simulink model "CostFunctionTuning"  (R2025b)
settings: Solver=FixedStepAuto  StartTime=0.0  StopTime=10.0  FixedStep=0.5  RelTol=1e-3  EnableMultiTasking=on
undefined symbols (not defined in the file): finalPose, initialPose, samplingBoxCenterPose, samplingBoxDimension, verticesStaticObstacles
libraries: MPSV x3
settings Model: Creator=Scythe  LastModifiedBy=Scythe
settings SolverCC: ConcurrentTasks=on
settings DataIOCC: SaveOutput=off  SignalLogging=off  DSMLogging=off  SaveTime=off  ReturnWorkspaceOutputs=off
settings OptimizationCC: DefaultParameterBehavior=Inlined  ZeroExternalMemoryAtStartup=off  ZeroInternalMemoryAtStartup=off  SimCompilerOptimization=on
settings DebuggingCC: UnconnectedInputMsg=warning  UnconnectedOutputMsg=warning  UnconnectedLineMsg=warning
settings HardwareCC: ProdBitPerLong=64.0  ProdHWDeviceType=Intel->x86-64 (Linux 64)  TargetBitPerLong=64.0  TargetBitPerPointer=64.0  TargetBitPerSizeT=64.0  TargetBitPerPtrDiffT=64.0  TargetLargestAtomicFloat=Float  TargetIntDivRoundTo=Zero  TargetEndianess=LittleEndian  TargetWordSize=64.0  TargetHWDeviceType=Intel->x86-64 (Linux 64)  ProdEqTarget=off
settings ModelReferenceCC: EnableRefExpFcnMdlSchedulingChecks=on
settings SFSimCC: SimParseCustomCode=off  SimGenImportedTypeDefs=on  SimTargetLang=C++  SimDLTargetLibrary=mkl-dnn
settings RTWCC: GenCodeOnly=on  PackageGeneratedCodeAndArtifacts=on  PackageName=PackNGo  BuildConfiguration=Faster Runs  TargetLang=C++
settings CodeAppCC: ForceParamTrailComments=on  MaxIdLength=128.0  StateflowObjectComments=on  MATLABSourceComments=on  UseSimReservedNames=on
settings GRTTargetCC: TargetLangStandard=C++11 (ISO)  MatFileLogging=off  CodeInterfacePackaging=C++ class  SubcomponentCodeInterfacePackaging=C++ class

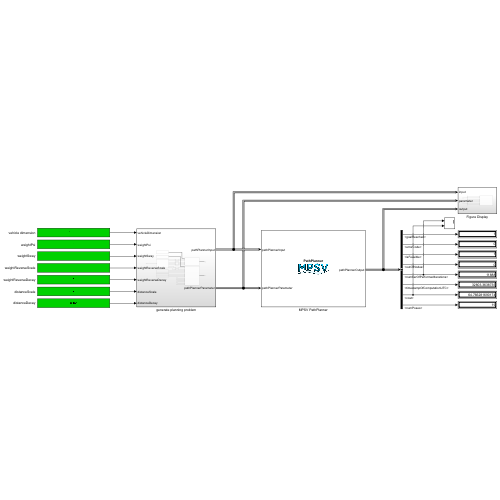
[thumbnail: Simulink's stored preview of the top-level diagram]
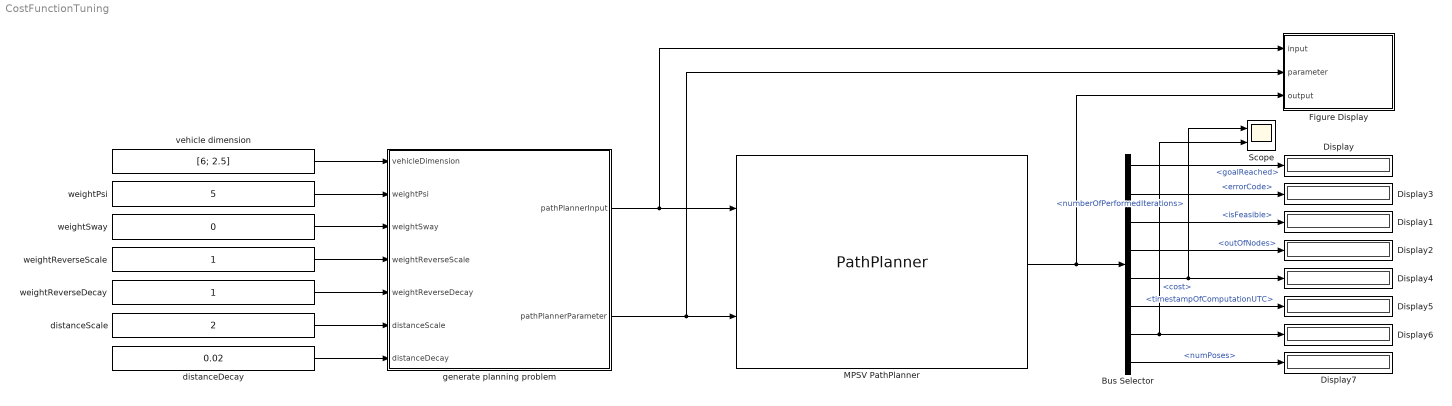
== system CostFunctionTuning ==
  Bus Selector : BusSelector  OutputSignals=goalReached,errorCode,isFeasible,outOfNodes,numberOfPerformedIterations,timestampOfComputationUTC,cost,numPoses
  Display{,1..7} (8 alike) : Display
  Figure Display : Subsystem
  MPSV PathPlanner : MPSV/PathPlanner  maxNumNodes=1000  maxNumSamples=1000000
      settings: SourceProductName=MPSV - Motion Planner for Surface Vehicles
  Scope : Scope  NumInputPorts=2
      settings: ActiveDisplayYMinimum=19472  ActiveDisplayYMaximum=20852
  distanceDecay : Constant  Value=0.02
  distanceScale : Constant  Value=2
  generate planning problem : Subsystem
  vehicle dimension : Constant  Value=[6; 2.5]
  weightPsi : Constant  Value=5
  weightReverseDecay : Constant
  weightReverseScale : Constant
  weightSway : Constant  Value=0
  wires:
  Bus Selector/5 -> Display4/1, Scope/1  "<numberOfPerformedIterations>"
  Bus Selector/6 -> Display5/1  "<timestampOfComputationUTC>"
  Bus Selector/7 -> Display6/1, Scope/2  "<cost>"
  Bus Selector/8 -> Display7/1  "<numPoses>"
  Bus Selector/2 -> Display3/1  "<errorCode>"
  Bus Selector/4 -> Display2/1  "<outOfNodes>"
  Bus Selector/3 -> Display1/1  "<isFeasible>"
  Bus Selector/1 -> Display/1  "<goalReached>"
  MPSV PathPlanner/1 -> Bus Selector/1, Figure Display/3(output)
  generate planning problem/2(pathPlannerParameter) -> Figure Display/2(parameter), MPSV PathPlanner/2
  generate planning problem/1(pathPlannerInput) -> MPSV PathPlanner/1, Figure Display/1(input)
  vehicle dimension/1 -> generate planning problem/1(vehicleDimension)
  weightPsi/1 -> generate planning problem/2(weightPsi)
  weightSway/1 -> generate planning problem/3(weightSway)
  weightReverseScale/1 -> generate planning problem/4(weightReverseScale)
  weightReverseDecay/1 -> generate planning problem/5(weightReverseDecay)
  distanceScale/1 -> generate planning problem/6(distanceScale)
  distanceDecay/1 -> generate planning problem/7(distanceDecay)

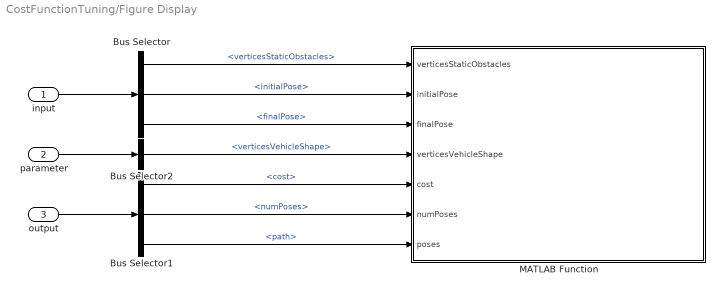
== system CostFunctionTuning/Figure Display ==
  input : Inport
  parameter : Inport  Port=2
  output : Inport  Port=3
  Bus Selector : BusSelector  OutputSignals=verticesStaticObstacles,initialPose,finalPose
  Bus Selector1 : BusSelector  OutputSignals=cost,numPoses,path
  Bus Selector2 : BusSelector  OutputSignals=geometry.verticesVehicleShape
  MATLAB Function : MATLAB Function  TreatAsAtomicUnit=on
  wires:
  Bus Selector2/1 -> MATLAB Function/4(verticesVehicleShape)  "<verticesVehicleShape>"
  Bus Selector1/3 -> MATLAB Function/7(poses)  "<path>"
  Bus Selector1/2 -> MATLAB Function/6(numPoses)  "<numPoses>"
  Bus Selector1/1 -> MATLAB Function/5(cost)  "<cost>"
  output/1 -> Bus Selector1/1
  Bus Selector/3 -> MATLAB Function/3(finalPose)  "<finalPose>"
  Bus Selector/2 -> MATLAB Function/2(initialPose)  "<initialPose>"
  Bus Selector/1 -> MATLAB Function/1(verticesStaticObstacles)  "<verticesStaticObstacles>"
  input/1 -> Bus Selector/1
  parameter/1 -> Bus Selector2/1

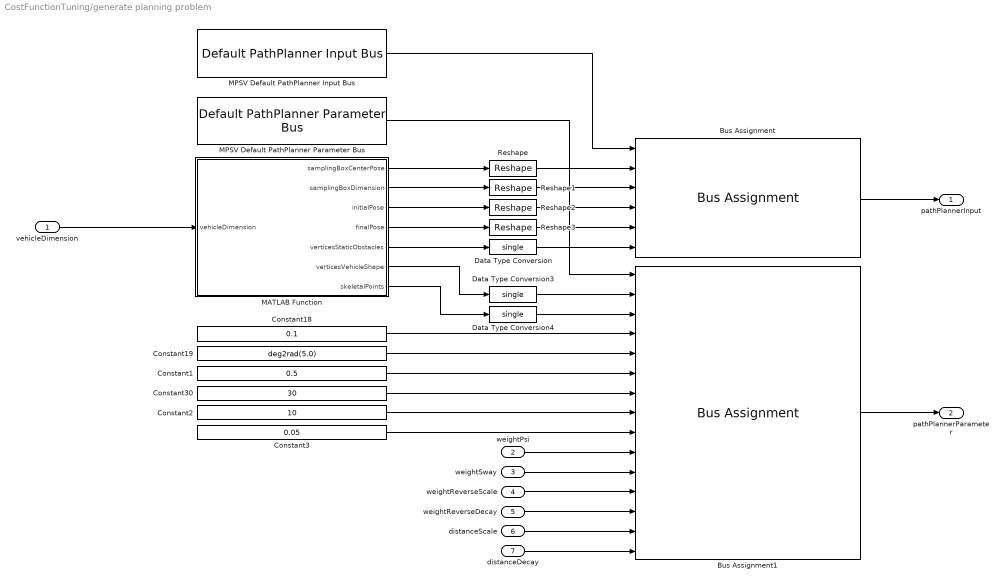
== system CostFunctionTuning/generate planning problem ==
  vehicleDimension : Inport
  weightPsi : Inport  Port=2
  weightSway : Inport  Port=3
  weightReverseScale : Inport  Port=4
  weightReverseDecay : Inport  Port=5
  distanceScale : Inport  Port=6
  distanceDecay : Inport  Port=7
  Bus Assignment : BusAssignment  AssignedSignals=samplingBoxCenterPose,samplingBoxDimension,initialPose,finalPose,verticesStaticObstacles
  Bus Assignment1 : BusAssignment  AssignedSignals=geometry.verticesVehicleShape,geometry.skeletalPoints,geometry.collisionCheckMaxPositionDeviation,geometry.collisionCheckMaxAngleDeviation,pathPlanner.maxComputationTime,pathPlanner.periodGoalSampling,costMap.modBreakpoints,costMap.resolution,metric.weightPsi,metric.weightSway,metric.weightReverseScale,metric.weightReverseDecay,costMap.distanceScale,costMap.distanceDecay
  Constant1 : Constant  Value=0.5
  Constant18 : Constant  Value=0.1  OutDataTypeStr=double
  Constant19 : Constant  Value=deg2rad(5.0)  OutDataTypeStr=double
  Constant2 : Constant  Value=10  OutDataTypeStr=int32
  Constant3 : Constant  Value=0.05  OutDataTypeStr=double
  Constant30 : Constant  Value=30  OutDataTypeStr=uint32
  Data Type Conversion : DataTypeConversion  OutDataTypeStr=single  SaturateOnIntegerOverflow=off  RndMeth=Floor
  Data Type Conversion3 : DataTypeConversion  OutDataTypeStr=single  SaturateOnIntegerOverflow=off  RndMeth=Floor
  Data Type Conversion4 : DataTypeConversion  OutDataTypeStr=single  SaturateOnIntegerOverflow=off  RndMeth=Floor
  MATLAB Function : MATLAB Function  TreatAsAtomicUnit=on
  MPSV Default PathPlanner Input Bus : MPSV/Default PathPlanner Input Bus
      settings: SourceProductName=MPSV - Motion Planner for Surface Vehicles
  MPSV Default PathPlanner Parameter Bus : MPSV/Default PathPlanner Parameter Bus
      settings: SourceProductName=MPSV - Motion Planner for Surface Vehicles
  Reshape{,1..3} (4 alike) : Reshape
  pathPlannerInput : Outport
  pathPlannerParameter : Outport  Port=2
  wires:
  MATLAB Function/2(samplingBoxDimension) -> Reshape1/1
  Constant19/1 -> Bus Assignment1/5
  Data Type Conversion/1 -> Bus Assignment/6
  weightPsi/1 -> Bus Assignment1/10
  MPSV Default PathPlanner Parameter Bus/1 -> Bus Assignment1/1
  distanceScale/1 -> Bus Assignment1/14
  Constant18/1 -> Bus Assignment1/4
  Data Type Conversion3/1 -> Bus Assignment1/2
  Constant1/1 -> Bus Assignment1/6
  MPSV Default PathPlanner Input Bus/1 -> Bus Assignment/1
  Data Type Conversion4/1 -> Bus Assignment1/3
  Constant2/1 -> Bus Assignment1/8
  Bus Assignment1/1 -> pathPlannerParameter/1
  MATLAB Function/6(verticesVehicleShape) -> Data Type Conversion3/1
  MATLAB Function/1(samplingBoxCenterPose) -> Reshape/1
  MATLAB Function/3(initialPose) -> Reshape2/1
  distanceDecay/1 -> Bus Assignment1/15
  MATLAB Function/5(verticesStaticObstacles) -> Data Type Conversion/1
  MATLAB Function/4(finalPose) -> Reshape3/1
  Constant3/1 -> Bus Assignment1/9
  MATLAB Function/7(skeletalPoints) -> Data Type Conversion4/1
  Constant30/1 -> Bus Assignment1/7
  vehicleDimension/1 -> MATLAB Function/1(vehicleDimension)
  weightReverseDecay/1 -> Bus Assignment1/13
  Bus Assignment/1 -> pathPlannerInput/1
  weightSway/1 -> Bus Assignment1/11
  weightReverseScale/1 -> Bus Assignment1/12
  Reshape/1 -> Bus Assignment/2
  Reshape1/1 -> Bus Assignment/3
  Reshape2/1 -> Bus Assignment/4
  Reshape3/1 -> Bus Assignment/5

== matlab function CostFunctionTuning/generate planning problem/MATLAB Function ==
  data: samplingBoxCenterPose output; samplingBoxDimension output; initialPose output; finalPose output; verticesStaticObstacles output; vehicleDimension input; verticesVehicleShape output; skeletalPoints output
function [samplingBoxCenterPose, samplingBoxDimension, initialPose, finalPose, verticesStaticObstacles, verticesVehicleShape, skeletalPoints]  = fcn(vehicleDimension)
    x = vehicleDimension(1) / 2;
    y = vehicleDimension(2) / 2;
    verticesVehicleShape = [[x -x -x x; y y -y -y], nan(2,96)];
    [skeletalPoints, ~] = mpsv.designer.details.BuildSkeletalPoints(verticesVehicleShape);
    samplingBoxCenterPose = [0;0;0];
    samplingBoxDimension = [10; 10] * max(vehicleDimension);
    initialPose = [-4 * max(vehicleDimension); 0; 0];
    finalPose = [4 * max(vehicleDimension); 0; deg2rad(90)];
    verticesStaticObstacles = [[2 -2 -1 1; 2 2 0 0] * max(vehicleDimension), nan(2,8000-4)];
end

== matlab function CostFunctionTuning/Figure Display/MATLAB Function ==
  data: verticesStaticObstacles input; initialPose input; finalPose input; verticesVehicleShape input; cost input; numPoses input; poses input
function FigureDisplay(verticesStaticObstacles, initialPose, finalPose, verticesVehicleShape, cost, numPoses, poses)
    persistent f;
    if(isempty(f))
        f = figure(42);
    end

    clf;
    hold on;
    PlotPath(numPoses, poses, verticesVehicleShape, [0 0.3 0.5]);
    PlotVehicleShape(initialPose, verticesVehicleShape, [0.9 0 0]);
    PlotVehicleShape(finalPose, verticesVehicleShape, [0 0.7 0]);
    PlotObstacles(verticesStaticObstacles);
    view(90,-90);
    axis equal;
    box on;
    grid on;
    xlabel('x in m');
    ylabel('y in m');
    title(sprintf('cost: %f',cost));
    drawnow();
end

function PlotPath(numPoses, poses, verticesVehicleShape, color)
    x = poses(1,1:numPoses);
    y = poses(2,1:numPoses);
    plot(x,y,'LineWidth',2,'Color',color);
    for i = uint32(1):uint32(numPoses)
        PlotVehicleShape(poses(:,i), verticesVehicleShape, color);
    end
end

function PlotVehicleShape(pose, verticesVehicleShape, color)
    c = cos(pose(3));
    s = sin(pose(3));
    R = [c -s; s c];

    N = int32(size(verticesVehicleShape,2));
    i0 = int32(-1);

    for i = int32(1):N
        finiteVertex = isfinite(verticesVehicleShape(1,i)) && isfinite(verticesVehicleShape(2,i));
        if((i0 < 1) && finiteVertex)
            i0 = i;
        elseif((i0 > 0) && (~finiteVertex || (i == N)))
            i = i + int32((i == N) && finiteVertex);
            vertices = R * verticesVehicleShape(:,i0:(i-1)) + [pose(1); pose(2)];
            PlotPolygon(vertices, color);
            plot(pose(1),pose(2),'o','Color',color);
            i0 = int32(-1);
        end
    end
end

function PlotObstacles(verticesStaticObstacles)
    N = int32(size(verticesStaticObstacles,2));
    i0 = int32(-1);

    for i = int32(1):N
        finiteVertex = isfinite(verticesStaticObstacles(1,i)) && isfinite(verticesStaticObstacles(2,i));
        if((i0 < 1) && finiteVertex)
            i0 = i;
        elseif((i0 > 0) && (~finiteVertex || (i == N)))
            i = i + int32((i == N) && finiteVertex);
            PlotPolygon(verticesStaticObstacles(:,i0:(i-1)), [0,0,0]);
            i0 = int32(-1);
        end
    end
end

function PlotPolygon(vertices, color)
    x = [vertices(1,:) vertices(1,1)];
    y = [vertices(2,:) vertices(2,1)];
    plot(x,y,'LineWidth',1,'Color',color);
end
